simulink model "ec_gravity_compensation"  (R2022a)
settings: Solver=ode3  StartTime=0.0  StopTime=inf  FixedStep=0.05  RelTol=1e-3
libraries: EcBlockToolbox x2, EcUtilities x2, Utilities x1, XBotBlockToolbox x1

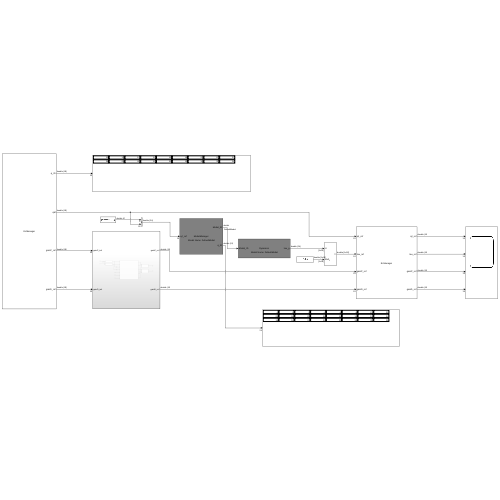
[thumbnail: Simulink's stored preview of the top-level diagram]
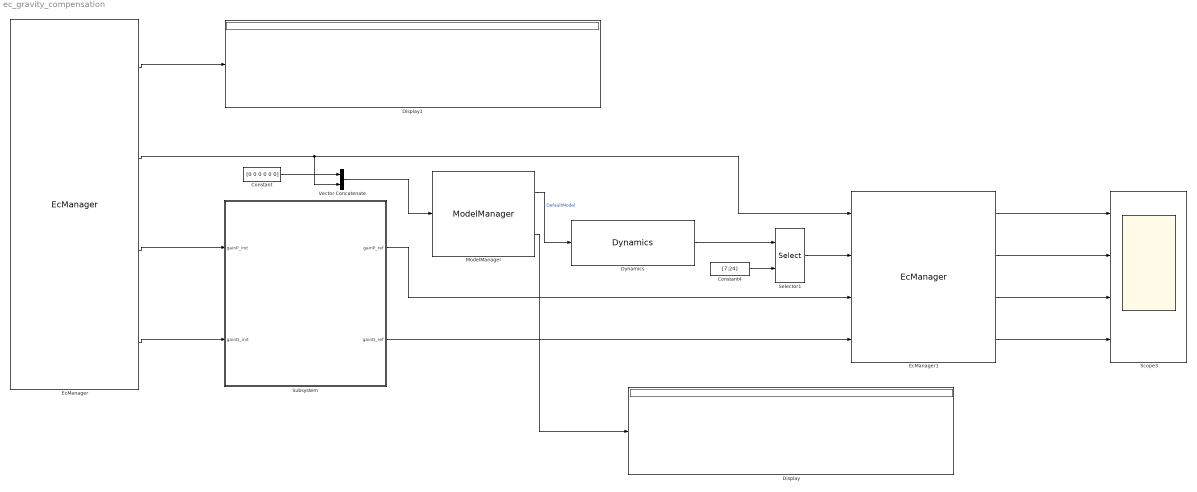
== system ec_gravity_compensation ==
  Constant : Constant  Value=[0 0 0 0 0 0]
  Constant4 : Constant  Value=[7:24]  VectorParams1D=off
  Display : Display
  Display1 : Display
  Dynamics : Utilities/Dynamics  ModelName=DefaultModel  ComponentsList={ 'tau_g' }
  EcManager : EcBlockToolbox/EcManager  PowList={}  ReadingsList={'q_ID', 'qM', 'gainP_ref', 'gainD_ref'}  ReferencesList={}  ImuList={}  FtList={}
  EcManager1 : EcBlockToolbox/EcManager  PowList={}  ReadingsList={'qJ_ref', 'tau_ref', 'gainP_ref', 'gainD_ref'}  ReferencesList={'qJ_ref', 'tau_ref', 'gainP_ref', 'gainD_ref'}  ImuList={}  FtList={}
  ModelManager : XBotBlockToolbox/ModelManager  ModelName=DefaultModel  RobotName=DefaultRobot  UseExtModel=Off  SyncWithRobot=Off  GetFloatingBaseList={}  SetFloatingBaseComponent=Off  GravityRequest=Off  ReadingsList={'q_ID'}  MechanicalLimitsList={}  MechanicalLimitsCheck=Off  MechanicalLimitsEnforce=Off  SensorList={}  ReferencesList={'qJ_ref'}  OldModelName=DefaultModel
  Scope3 : Scope  NumInputPorts=4
  Selector1 : Selector  NumberOfDimensions=2  IndexOptions=Select all,Index vector (port)  Indices=[1 3],1  OutputSizes=1,1
  Subsystem : Subsystem
  Vector Concatenate : Concatenate
  wires:
  EcManager1/1 -> Scope3/1
  EcManager1/2 -> Scope3/2
  EcManager1/3 -> Scope3/3
  Subsystem/1(gainP_ref) -> EcManager1/3
  Subsystem/2(gainD_ref) -> EcManager1/4
  ModelManager/1 -> Dynamics/1  "DefaultModel"
  EcManager/2 -> Vector Concatenate/2, EcManager1/1
  ModelManager/2 -> Display/1
  EcManager/3 -> Subsystem/1(gainP_init)
  EcManager/4 -> Subsystem/2(gainD_init)
  Constant/1 -> Vector Concatenate/1
  Vector Concatenate/1 -> ModelManager/1
  EcManager/1 -> Display1/1
  Selector1/1 -> EcManager1/2
  Dynamics/1 -> Selector1/1
  Constant4/1 -> Selector1/2
  EcManager1/4 -> Scope3/4

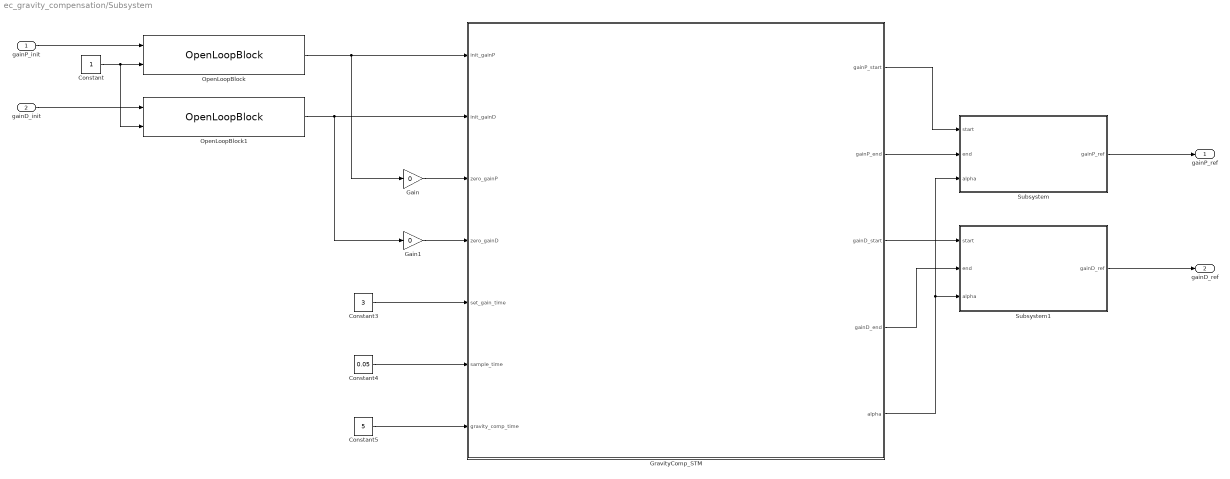
== system ec_gravity_compensation/Subsystem ==
  gainP_init : Inport
  gainD_init : Inport  Port=2
  Constant : Constant
  Constant3 : Constant  Value=3
  Constant4 : Constant  Value=0.05
  Constant5 : Constant  Value=5
  Gain : Gain  Gain=0
  Gain1 : Gain  Gain=0
  GravityComp_STM : Stateflow chart  TreatAsAtomicUnit=on
  OpenLoopBlock : EcUtilities/OpenLoopBlock  SystemSampleTime=-1  VariantActivationTime=update diagram  Latency=0  AutoFrameSizeCalculation=off
  OpenLoopBlock1 : EcUtilities/OpenLoopBlock  SystemSampleTime=-1  VariantActivationTime=update diagram  Latency=0  AutoFrameSizeCalculation=off
  Subsystem : Subsystem
  Subsystem1 : Subsystem
  gainP_ref : Outport
  gainD_ref : Outport  Port=2
  wires:
  Constant5/1 -> GravityComp_STM/7(gravity_comp_time)
  OpenLoopBlock1/1 -> Gain1/1, GravityComp_STM/2(init_gainD)
  GravityComp_STM/5(alpha) -> Subsystem/3(alpha), Subsystem1/3(alpha)
  Constant4/1 -> GravityComp_STM/6(sample_time)
  gainP_init/1 -> OpenLoopBlock/1
  Subsystem/1(gainP_ref) -> gainP_ref/1
  OpenLoopBlock/1 -> Gain/1, GravityComp_STM/1(init_gainP)
  Constant/1 -> OpenLoopBlock/2, OpenLoopBlock1/2
  gainD_init/1 -> OpenLoopBlock1/1
  Gain/1 -> GravityComp_STM/3(zero_gainP)
  Gain1/1 -> GravityComp_STM/4(zero_gainD)
  Constant3/1 -> GravityComp_STM/5(set_gain_time)
  Subsystem1/1(gainD_ref) -> gainD_ref/1
  GravityComp_STM/2(gainP_end) -> Subsystem/2(end)
  GravityComp_STM/4(gainD_end) -> Subsystem1/2(end)
  GravityComp_STM/1(gainP_start) -> Subsystem/1(start)
  GravityComp_STM/3(gainD_start) -> Subsystem1/1(start)

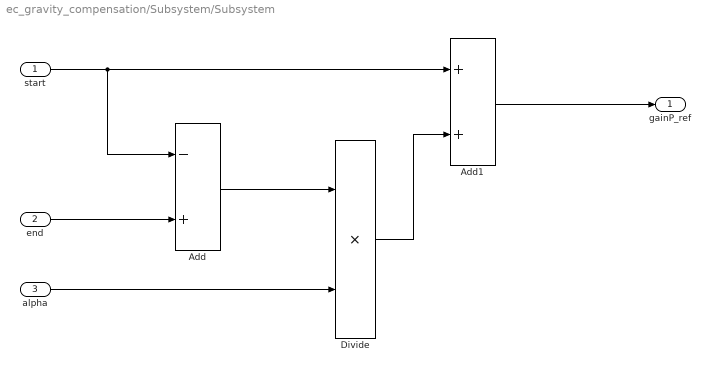
== system ec_gravity_compensation/Subsystem/Subsystem ==
  start : Inport
  end : Inport  Port=2
  alpha : Inport  Port=3
  Add : Sum  Inputs=-+
  Add1 : Sum
  Divide : Product  Inputs=**
  gainP_ref : Outport
  wires:
  Divide/1 -> Add1/2
  Add/1 -> Divide/1
  start/1 -> Add1/1, Add/1
  end/1 -> Add/2
  alpha/1 -> Divide/2
  Add1/1 -> gainP_ref/1

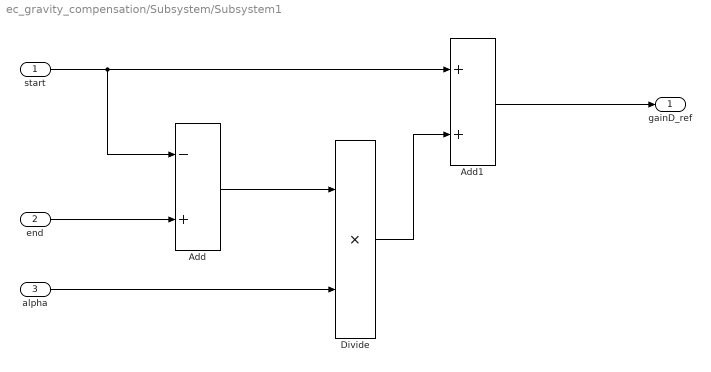
== system ec_gravity_compensation/Subsystem/Subsystem1 ==
  start : Inport
  end : Inport  Port=2
  alpha : Inport  Port=3
  Add : Sum  Inputs=-+
  Add1 : Sum
  Divide : Product  Inputs=**
  gainD_ref : Outport
  wires:
  Divide/1 -> Add1/2
  Add/1 -> Divide/1
  start/1 -> Add1/1, Add/1
  end/1 -> Add/2
  alpha/1 -> Divide/2
  Add1/1 -> gainD_ref/1

== stateflow chart ec_gravity_compensation/Subsystem/GravityComp_STM ==
  state Motor_Ctrl_SetGains_Zero
    en: gainP_end = zero_gainP; gainD_end=zero_gainD; gainP_start = init_gainP; gainD_start=init_gainD; time=0;alpha=0;
    du: time=time + sample_time;
    tau=time/set_gain_time;
    alpha = ((6*tau - 15)*tau + 10)*tau*tau*tau;
  state Motor_Ctrl_Gravity
    en: time=0;
    du: time=time + sample_time;
  state Motor_Ctrl_SetGains_InitValue
    en: gainP_end = init_gainP; gainD_end=init_gainD; gainP_start = zero_gainP; gainD_start=zero_gainD; time=0;alpha=0;
    du: time=time + sample_time;
    tau=time/set_gain_time;
    alpha = ((6*tau - 15)*tau + 10)*tau*tau*tau;
  state Stop
  (default) -> Motor_Ctrl_SetGains_Zero
  Motor_Ctrl_SetGains_Zero -> Motor_Ctrl_Gravity : [time >= set_gain_time]
  Motor_Ctrl_Gravity -> Motor_Ctrl_SetGains_InitValue : [time >= gravity_comp_time]
  Motor_Ctrl_SetGains_InitValue -> Stop : [time >= set_gain_time]
  data: gainP_start output; gainP_end output; gainD_start output; init_gainP input; init_gainD input; gainD_end output; zero_gainP input; zero_gainD input; set_gain_time input; sample_time input; gravity_comp_time input; time local =0; alpha output; tau local =0
